simulink library "tetherSpeedController"  (R2018a)
settings: Solver=VariableStepAuto  StartTime=0.0  StopTime=10.0  RelTol=1e-3
undefined symbols (not defined in the file): iterationPhase_enum
libraries: calculateReelInSpeed x1, calculateReelOutSpeed x1, simulink x1
settings Model: Creator=mitch  LastModifiedBy=mitch

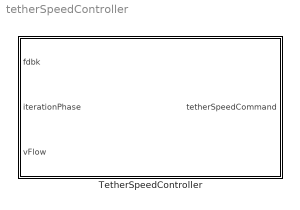
== system tetherSpeedController ==
  TetherSpeedController : Subsystem

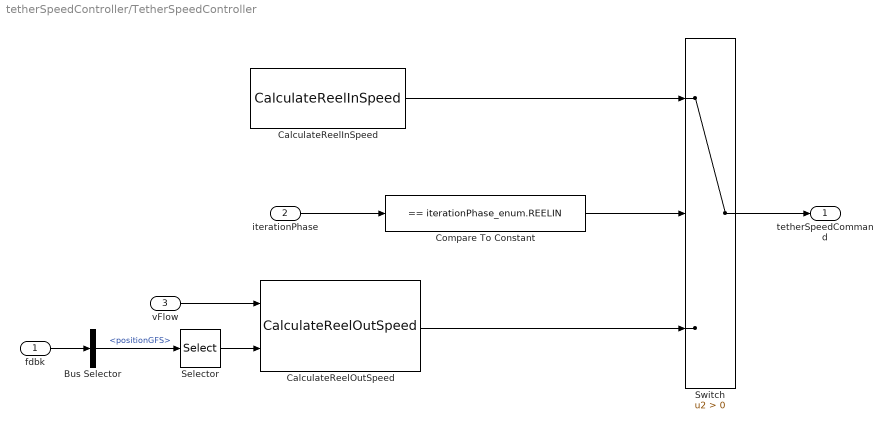
== system tetherSpeedController/TetherSpeedController ==
  fdbk : Inport  OutDataTypeStr=Bus: busPlantFeedback
  iterationPhase : Inport  Port=2
  vFlow : Inport  Port=3
  Bus Selector : BusSelector  OutputSignals=positionGFS
  CalculateReelInSpeed : calculateReelInSpeed/CalculateReelInSpeed
  CalculateReelOutSpeed : calculateReelOutSpeed/CalculateReelOutSpeed
  Compare To Constant : simulink/Logic and Bit Operations/Compare To Constant  relop===  const=iterationPhase_enum.REELIN  OutDataTypeStr=boolean
  Selector : Selector  InputPortWidth=3  IndexOptions=Index vector (dialog)  Indices=3  OutputSizes=1
  Switch : Switch  Criteria=u2 > Threshold
  tetherSpeedCommand : Outport
  wires:
  vFlow/1 -> CalculateReelOutSpeed/1
  CalculateReelInSpeed/1 -> Switch/1
  CalculateReelOutSpeed/1 -> Switch/3
  Switch/1 -> tetherSpeedCommand/1
  fdbk/1 -> Bus Selector/1
  Bus Selector/1 -> Selector/1  "<positionGFS>"
  Selector/1 -> CalculateReelOutSpeed/2
  iterationPhase/1 -> Compare To Constant/1
  Compare To Constant/1 -> Switch/2
